simulink model "readMessageTest"  (R2017a)
settings: Solver=FixedStepAuto  StartTime=0.0  StopTime=inf  FixedStep=.004  RelTol=1e-3
model workspace (MAT data in the model file):
  SL_ROS_VariableLengthArrays_MaxSizes.CommonInfo.ArrayTruncateAction = 'EmitWarning'
  SL_ROS_VariableLengthArrays_MaxSizes.MsgTypeMap = containers.Map
  SL_ROS_VariableLengthArrays_MaxSizes.MsgTypeMap.serialization.keys = {'std_msgs/Int16MultiArray'}
  SL_ROS_VariableLengthArrays_MaxSizes.MsgTypeMap.serialization.values{1}.PropertyName = 'Data'
  SL_ROS_VariableLengthArrays_MaxSizes.MsgTypeMap.serialization.values{1}.DataType = 'int16'
  SL_ROS_VariableLengthArrays_MaxSizes.MsgTypeMap.serialization.values{1}.MaxLength = 2
  SL_ROS_VariableLengthArrays_MaxSizes.MsgTypeMap.serialization.uniformity = 0
  SL_ROS_VariableLengthArrays_MaxSizes.MsgTypeMap.serialization.keyType = 'char'
  SL_ROS_VariableLengthArrays_MaxSizes.MsgTypeMap.serialization.valueType = 'any'
undefined symbols (not defined in the file or in its folder): A_butter_low, B_butter_low
libraries: robotlib x3
settings Model: Creator=jacob  LastModifiedBy=jacob

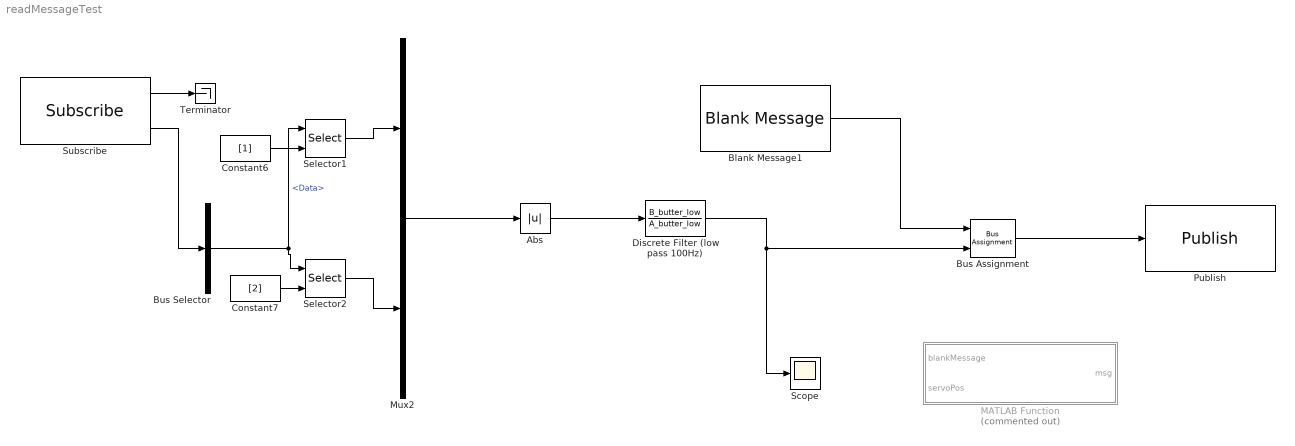
== system readMessageTest ==
  Abs : Abs
  Blank Message1 : robotlib/Blank Message  SourceLibraryInfo=This block requires Robotics System Toolbox  messageType=std_msgs/Int16MultiArray  SampleTime=inf
      settings: SourceProductBaseCode=RO
  Bus Assignment : BusAssignment  AssignedSignals=Data
  Bus Selector : BusSelector  OutputSignals=Data
  Constant6 : Constant  Value=[1]
  Constant7 : Constant  Value=[2]
  Discrete Filter (low pass 100Hz) : DiscreteFilter  Numerator=B_butter_low  Denominator=A_butter_low
  MATLAB Function : MATLAB Function  Commented=on  TreatAsAtomicUnit=on
  Mux2 : Mux  Inputs=2
  Publish : robotlib/Publish  SourceLibraryInfo=This block requires Robotics System Toolbox  topicSource=Specify your own  topic=/blah  messageType=std_msgs/Int16MultiArray  messageQueueLength=1
      settings: SourceProductBaseCode=RO
  Scope : Scope
  Selector1 : Selector  IndexOptions=Index vector (port)  Indices=[1 3]  OutputSizes=1
  Selector2 : Selector  IndexOptions=Index vector (port)  Indices=[1 3]  OutputSizes=1
  Subscribe : robotlib/Subscribe  SourceLibraryInfo=This block requires Robotics System Toolbox  topicSource=Select from ROS network  topic=/emgPub  messageType=std_msgs/Int16MultiArray  sampleTime=-1  messageQueueLength=1
      settings: SourceProductBaseCode=RO
  Terminator : Terminator
  wires:
  Subscribe/1 -> Terminator/1
  Constant7/1 -> Selector2/2
  Bus Selector/1 -> Selector2/1, Selector1/1  "<Data>"
  Abs/1 -> Discrete Filter (low pass 100Hz)/1
  Selector1/1 -> Mux2/1
  Subscribe/2 -> Bus Selector/1
  Constant6/1 -> Selector1/2
  Mux2/1 -> Abs/1
  Discrete Filter (low pass 100Hz)/1 -> Bus Assignment/2, Scope/1
  Bus Assignment/1 -> Publish/1
  Blank Message1/1 -> Bus Assignment/1
  Selector2/1 -> Mux2/2

== matlab function readMessageTest/MATLAB Function ==
  data: blankMessage input; servoPos input; msg output Bus: <blankMessage>
function msg = createMessage(blankMessage,servoPos)
robotics.ros.createSimulinkBus(gcs)

blankMessage.layout.dim[0].size = 2;
blankMessage.layout.dim[0].stride = 1*2;
blankMessage.data_length = 2;
blankMessage.data = servoPos;

msg = blankMessage;
% end function
